simulink subsystem "AnalyticInverseFourBarLinkage"  (R2020b)
settings: Solver=VariableStepAuto  StartTime=0.0  StopTime=10.0  RelTol=1e-3
model mask{g=21, a=10.17, h=30.625, b=20.78, solutionSelector=1}
  mask prompts: g "g Distance between pivots"; a "a Length of crank arm"; h "h Length of coupler arm"; b "b Length of rocker arm"; solutionSelector "Solution number (1 or 2)"
settings Model: Creator=Edward  LastModifiedBy=Edward

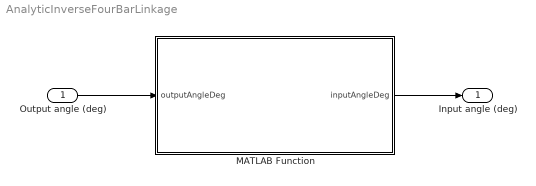
== system AnalyticInverseFourBarLinkage ==
  Output angle (deg) : Inport
  MATLAB Function : MATLAB Function  TreatAsAtomicUnit=on
  Input angle (deg) : Outport
  wires:
  MATLAB Function/1(inputAngleDeg) -> Input angle (deg)/1
  Output angle (deg)/1 -> MATLAB Function/1(outputAngleDeg)

== matlab function AnalyticInverseFourBarLinkage/MATLAB Function ==
  data: outputAngleDeg input; inputAngleDeg output; g parameter; b parameter; a parameter; h parameter; solutionSelector parameter
%g, b, a, h, solutionSelector are params from the sim (See "Edit Data"
%button in ribbon)
function inputAngleDeg = getInputAngle(outputAngleDeg, g, b, a, h, solutionSelector)
assert(solutionSelector==1 || solutionSelector==2, "Solution selector must be 1 or 2");
inputAngleDegs = Mechanical.FourBarLinkage.getPossibleAnglesOfLeftLinkageDegrees(g, b, a, h, outputAngleDeg);

inputAngleDeg = inputAngleDegs(solutionSelector);
end
